simulink model "Modelagem_Foguete (1)"  (R2023a)
settings: Solver=VariableStepAuto  StartTime=0.0  StopTime=252  RelTol=1e-3
libraries: aerolibatmos2 x2
settings Model: Creator=pedro  LastModifiedBy=mluser
settings OptimizationCC: ReuseModelBlockBuffer=off

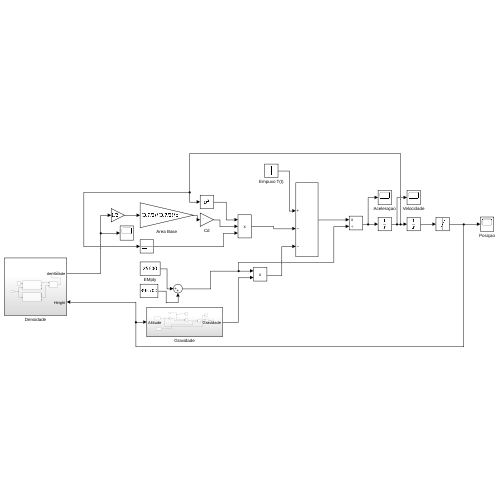
[thumbnail: Simulink's stored preview of the top-level diagram]
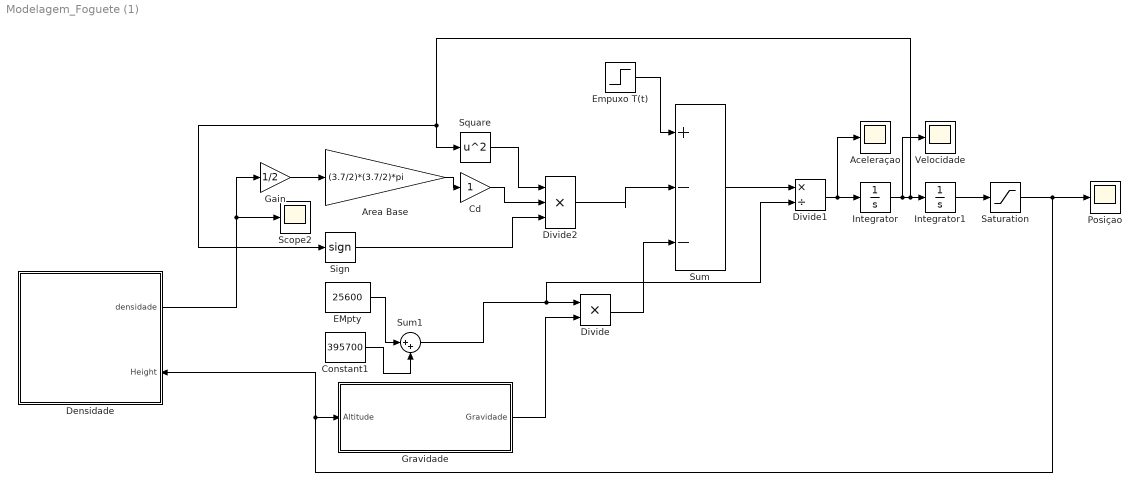
== system Modelagem_Foguete (1) ==
  Aceleraçao : Scope
  Area Base : Gain  Gain=(3.7/2)*(3.7/2)*pi
  Cd : Gain
  Constant1 : Constant  Value=395700
  Densidade : Subsystem
      settings: PortSchema="{\"entries\":[{\"content\":{\"sides\":[{\"content\":{},\"type\":\"ConnectorPlacement.EquallySpacedRectSide\",\"uuid\":\"1cd91c1d-e3da-4072-b1d5-bde77eaa4d77\"},{\"content\":{\"connectorIds\":[\"Out1\",\"In1\"],\"side\":\"RIGHT\"},\"type\":\"ConnectorPlacement.EquallySpacedRectSide\",\"uuid\":\"15adf8d6-6e17-4f5d-b81f-b315088c5251\"},{\"content\":{\"side\":\"TOP\"},\"type\":\"ConnectorPlacement.EquallySpacedRectSide\",\"uuid\":\"e4b32ce3-cb0a-46b5-82b1-bf4ba8b7d084\"}]},\"type\":\"ConnectorPlacement.EquallySpacedConnector\",\"uuid\":\"c32abf6f-6c50-4b1c-8a6c-37657812f68f\"}],\"packageUris\":[\"http://schema.mathworks.com/mf0/Connector/R2020b\"],\"version\":\"1.0\"}"
  Divide : Product  Inputs=**
  Divide1 : Product  Inputs=*/
  Divide2 : Product  Inputs=***
  EMpty : Constant  Value=25600
  Empuxo T(t) : Step  After=0  SampleTime=0
  Gain : Gain  Gain=1/2
  Gravidade : Subsystem
  Integrator : Integrator
  Integrator1 : Integrator  InitialCondition=127*1000
  Posiçao : Scope
  Saturation : Saturate  UpperLimit=inf  LowerLimit=0
  Scope2 : Scope
  Sign : Signum
  Square : Math  Operator=square
  Sum : Sum  Inputs=|+--
  Sum1 : Sum  Inputs=|++
  Velocidade : Scope
  wires:
  Empuxo T(t)/1 -> Sum/1
  Gravidade/1(Gravidade) -> Divide/2
  Divide/1 -> Sum/3
  Sum1/1 -> Divide1/2, Divide/1
  Sum/1 -> Divide1/1
  Divide1/1 -> Aceleraçao/1, Integrator/1
  Integrator/1 -> Velocidade/1, Square/1, Sign/1, Integrator1/1
  Square/1 -> Divide2/1
  Cd/1 -> Divide2/2
  Sign/1 -> Divide2/3
  Divide2/1 -> Sum/2
  Gain/1 -> Area Base/1
  Area Base/1 -> Cd/1
  EMpty/1 -> Sum1/1
  Constant1/1 -> Sum1/2
  Integrator1/1 -> Saturation/1
  Saturation/1 -> Densidade/1(Height), Gravidade/1(Altitude), Posiçao/1
  Densidade/1(densidade) -> Gain/1, Scope2/1

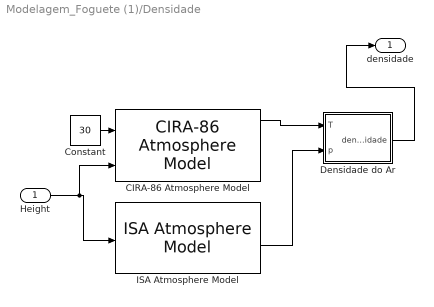
== system Modelagem_Foguete (1)/Densidade ==
  Height : Inport
  CIRA-86 Atmosphere Model : aerolibatmos2/CIRA-86 Atmosphere Model  units=Metric (MKS)  ctype=GPHeight  mtype=Monthly  month=June  action=Warning
  Constant : Constant  Value=30
  Densidade do Ar : Subsystem
  ISA Atmosphere Model : aerolibatmos2/ISA Atmosphere Model  custom=off  g=9.80665  gamma=1.4  R=287.0531  L=0.0065  h_trop=11000  h_strat=20000  rho0=1.225  P0=101325  T0=288.15  h0=0
  densidade : Outport
  wires:
  ISA Atmosphere Model/3 -> Densidade do Ar/2(p)
  Constant/1 -> CIRA-86 Atmosphere Model/1
  Height/1 -> CIRA-86 Atmosphere Model/2, ISA Atmosphere Model/1
  CIRA-86 Atmosphere Model/1 -> Densidade do Ar/1(T)
  Densidade do Ar/1(densidade) -> densidade/1

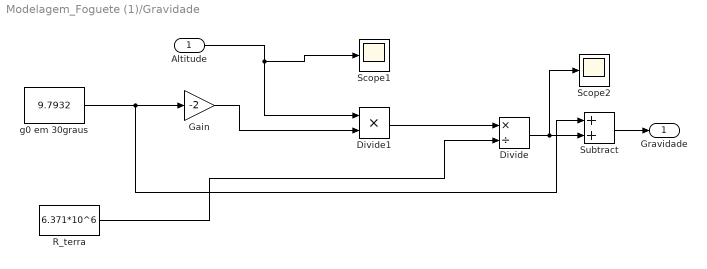
== system Modelagem_Foguete (1)/Gravidade ==
  Altitude : Inport
  Divide : Product  Inputs=*/
  Divide1 : Product  Inputs=**
  Gain : Gain  Gain=-2
  R_terra : Constant  Value=6.371*10^6
  Scope1 : Scope
  Scope2 : Scope
  Subtract : Sum
  g0 em 30graus : Constant  Value=9.7932
  Gravidade : Outport
  wires:
  g0 em 30graus/1 -> Subtract/1, Gain/1
  Gain/1 -> Divide1/2
  Subtract/1 -> Gravidade/1
  Divide/1 -> Scope2/1, Subtract/2
  Divide1/1 -> Divide/1
  R_terra/1 -> Divide/2
  Altitude/1 -> Scope1/1, Divide1/1

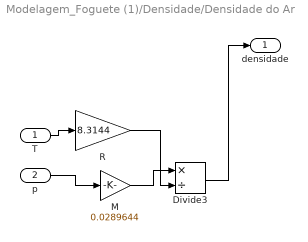
== system Modelagem_Foguete (1)/Densidade/Densidade do Ar ==
  T : Inport
  p : Inport  Port=2
  Divide3 : Product  Inputs=*/
  M : Gain  Gain=0.0289644
  R : Gain  Gain=8.3144
  densidade : Outport
  wires:
  R/1 -> Divide3/2
  M/1 -> Divide3/1
  p/1 -> M/1
  Divide3/1 -> densidade/1
  T/1 -> R/1
